simulink library "Driveline_Axle3_A2_A2Diff"  (R2026a)
settings: Solver=VariableStepAuto
libraries: Driveshaft_Assembly_None x4, sm_lib x2, Driveshaft_Assembly x2, Differential_Systems x1, fl_lib x1, sdl_lib x1
Description:
  | Component of Simscape Vehicle Templates Library
  | 
  | Copyright 2018-2026 The MathWorks, Inc.
settings Model: Creator=smiller  LastModifiedBy=smiller

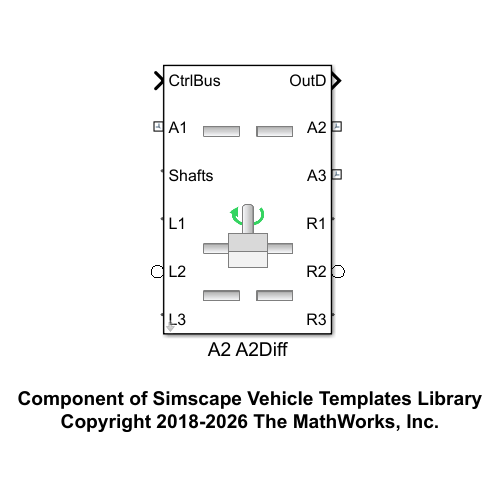
[thumbnail: Simulink's stored preview of the top-level diagram]
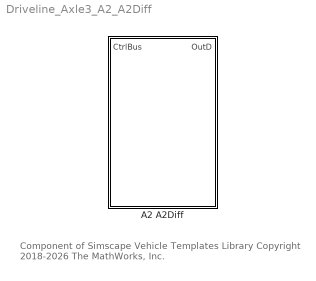
== system Driveline_Axle3_A2_A2Diff ==
  note: Component of Simscape Vehicle Templates Library
      | Copyright 2018-2026 The MathWorks, Inc.
  A2 A2Diff : Subsystem  Tag=PublishSubsystem  VariantControl=IndepFRDiffFDiffR  mask(Driveline 6x2, 3-Axle, One Input Shaft){}
      mask help: Models driveline with 3 axles. The second axle is powered by a single input shaft.
      mask Display: image('sm_car_vehicle_driveline_axle3_a2_a2diff_IMAGE.png');

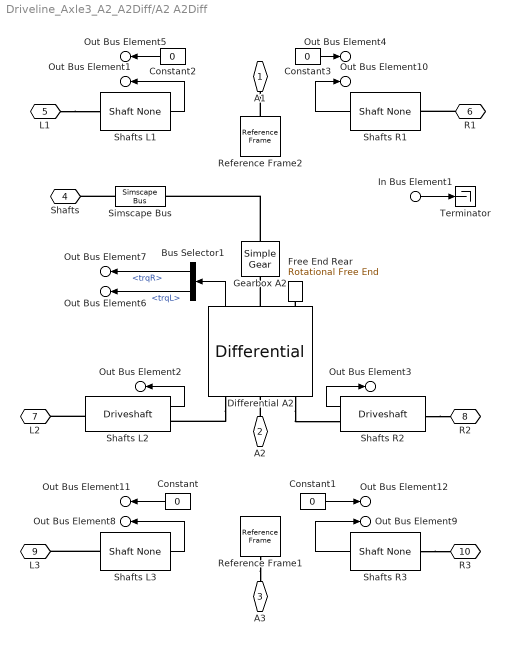
== system Driveline_Axle3_A2_A2Diff/A2 A2Diff ==
  In Bus Element1 : Inport  PortName=CtrlBus
  Bus Selector1 : BusSelector  OutputSignals=trqR,trqL
  Constant{,1..3} (4 alike) : Constant  Value=0
  Differential A2 : Differential_Systems/Differential  VariantControl=Variant1  LabelModeActiveChoice=Gear1DShafts1D  Differential=Driveline.DifferentialA2  VariantLabel=Driveline.DifferentialA2.class.Value
      settings: AttributesFormatString=%<ActiveVariant>
  Free End Rear : fl_lib/Mechanical/Rotational Elements/Rotational Free End  w_specify=off  w_priority=None  w=0 rad/s  w_nominal_specify=off  w_nominal_value=1  w_nominal_unit=rad/s
  Gearbox A2 : sdl_lib/Gears/Simple Gear  ratio=Driveline.GearboxA2.ratio.Value  rotation_direction=3-2*(1)  friction_model=1  T_noload=0.1 N*m  T_nom=5 N*m  efficiency_nom=0.8  efficiency=0.8  temperature_TLU=[280, 300, 320] K  load_TLU=[1, 5, 10] N*m  efficiency_TLU=[.95, .9, .85]  efficiency_TLU2=[.85, .8, .75; .95, .9, .85; .85, .8, .7]  w_thr=0.01 rad/s  pwr_thr=0.001 W  enable_backlash=false  hardstop_model=simscape.enum.hardstop.smooth  backlash_distance=1e-3 mm  r_base=0.1 m  transition=1e-4 mm  backlash_stiffness=1e7 N/m  backlash_damping=1e6 N*s/m  coeff_rest=0  v_tol=0.001 m/s  f_tol=0 N  tau=0.1 s  mu_visc=[0, 0] N*m/(rad/s)  thermal_mass=50 J/K  temperature_specify=off  temperature_priority=High  temperature=300 K  temperature_nominal_specify=off  temperature_nominal_value=1  temperature_nominal_unit=K  x_backlash_specify=off  x_backlash_priority=None  x_backlash=0 mm  x_backlash_nominal_specify=off  x_backlash_nominal_value=1  x_backlash_nominal_unit=mm  f_hardstop_specify=off  f_hardstop_priority=None  f_hardstop=0 N  f_hardstop_nominal_specify=off  f_hardstop_nominal_value=1  f_hardstop_nominal_unit=N  v_backlash_specify=off  v_backlash_priority=None  v_backlash=0 m/s  v_backlash_nominal_specify=off  v_backlash_nominal_value=1  v_backlash_nominal_unit=m/s
  Reference Frame1 : sm_lib/Frames and Transforms/Reference Frame
  Reference Frame2 : sm_lib/Frames and Transforms/Reference Frame
  Shafts L1 : Driveshaft_Assembly_None/Shaft None  VariantControl=Shaft1D
  Shafts L2 : Driveshaft_Assembly/Driveshaft  VariantControl=Variant1  LabelModeActiveChoice=Shaft1D  popup_leftRight=Left  Driveshaft=Driveline.DriveshaftL2  VariantLabel=Driveline.DriveshaftL2.class.Value
      settings: AttributesFormatString=%<ActiveVariant>
  Shafts L3 : Driveshaft_Assembly_None/Shaft None  VariantControl=Shaft1D
  Shafts R1 : Driveshaft_Assembly_None/Shaft None  VariantControl=Shaft1D
  Shafts R2 : Driveshaft_Assembly/Driveshaft  VariantControl=Variant1  LabelModeActiveChoice=Shaft1D  popup_leftRight=Right  Driveshaft=Driveline.DriveshaftR2  VariantLabel=Driveline.DriveshaftR2.class.Value
      settings: AttributesFormatString=%<ActiveVariant>
  Shafts R3 : Driveshaft_Assembly_None/Shaft None  VariantControl=Shaft1D
  Simscape Bus : SimscapeBus  HierarchyStrings=ShaftA2
  Terminator : Terminator
  A1 : PMIOPort  Side=Left
  A2 : PMIOPort  Port=2  Side=Right
  A3 : PMIOPort  Port=3  Side=Right
  Shafts : PMIOPort  Port=4  Side=Left
  L1 : PMIOPort  Port=5  Side=Left
  R1 : PMIOPort  Port=6  Side=Right
  L2 : PMIOPort  Port=7  Side=Left
  R2 : PMIOPort  Port=8  Side=Right
  L3 : PMIOPort  Port=9  Side=Left
  R3 : PMIOPort  Port=10  Side=Right
  Out Bus Element4 : Outport  VectorParamsAs1DForOutWhenUnconnected=off  PortName=OutD  Element=MDriveshaftR1
  Out Bus Element5 : Outport  VectorParamsAs1DForOutWhenUnconnected=off  PortName=OutD  Element=MDriveshaftL1
  Out Bus Element8 : Outport  VectorParamsAs1DForOutWhenUnconnected=off  PortName=OutD  Element=anDriveshaftL3
  Out Bus Element9 : Outport  VectorParamsAs1DForOutWhenUnconnected=off  PortName=OutD  Element=anDriveshaftR3
  Out Bus Element2 : Outport  VectorParamsAs1DForOutWhenUnconnected=off  PortName=OutD  Element=anDriveshaftL2
  Out Bus Element3 : Outport  VectorParamsAs1DForOutWhenUnconnected=off  PortName=OutD  Element=anDriveshaftR2
  Out Bus Element6 : Outport  VectorParamsAs1DForOutWhenUnconnected=off  PortName=OutD  Element=MDriveshaftL2
  Out Bus Element7 : Outport  VectorParamsAs1DForOutWhenUnconnected=off  PortName=OutD  Element=MDriveshaftR2
  Out Bus Element1 : Outport  VectorParamsAs1DForOutWhenUnconnected=off  PortName=OutD  Element=anDriveshaftL1
  Out Bus Element10 : Outport  VectorParamsAs1DForOutWhenUnconnected=off  PortName=OutD  Element=anDriveshaftR1
  Out Bus Element11 : Outport  VectorParamsAs1DForOutWhenUnconnected=off  PortName=OutD  Element=MDriveshaftL3
  Out Bus Element12 : Outport  VectorParamsAs1DForOutWhenUnconnected=off  PortName=OutD  Element=MDriveshaftR3
  wires:
  In Bus Element1/1 -> Terminator/1
  Shafts R3/1 -> Out Bus Element9/1
  Shafts L3/1 -> Out Bus Element8/1
  Shafts R2/1 -> Out Bus Element3/1
  Shafts L2/1 -> Out Bus Element2/1
  Differential A2/1 -> Bus Selector1/1
  Bus Selector1/1 -> Out Bus Element7/1  "<trqR>"
  Bus Selector1/2 -> Out Bus Element6/1  "<trqL>"
  Shafts L1/1 -> Out Bus Element1/1
  Shafts R1/1 -> Out Bus Element10/1
  Constant1/1 -> Out Bus Element12/1
  Constant/1 -> Out Bus Element11/1
  Constant2/1 -> Out Bus Element5/1
  Constant3/1 -> Out Bus Element4/1
  connections:
  Simscape Bus/RConn1 -- Shafts/RConn1
  Shafts L2/LConn1 -- L2/RConn1
  Shafts R2/LConn1 -- R2/RConn1
  Shafts R3/LConn1 -- R3/RConn1
  Reference Frame1/RConn1 -- A3/RConn1
  Shafts L3/LConn1 -- L3/RConn1
  A2/RConn1 -- Differential A2/LConn2
  Differential A2/LConn1 -- Shafts L2/RConn1
  Differential A2/LConn3 -- Shafts R2/RConn1
  Gearbox A2/LConn1 -- Simscape Bus/LConn1
  Differential A2/RConn2 -- Free End Rear/LConn1
  Differential A2/RConn1 -- Gearbox A2/RConn1
  L1/RConn1 -- Shafts L1/LConn1
  R1/RConn1 -- Shafts R1/LConn1
  Reference Frame2/RConn1 -- A1/RConn1
